simulink model "ModelReadWrite"  (R2016a)
settings: Solver=VariableStepAuto  StartTime=0.0  StopTime=30  RelTol=1e-3
libraries: ToolBox_Control_Lab x1
settings Model: Creator=steph  LastModifiedBy=steph

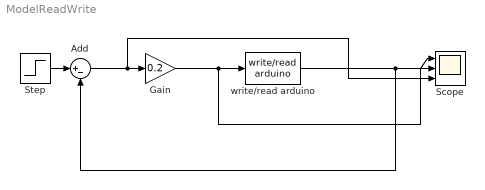
== system ModelReadWrite ==
  Add : Sum  Inputs=|+-
  Gain : Gain  Gain=0.2
  Scope : Scope  NumInputPorts=3
  Step : Step  Time=5  After=23  SampleTime=0
  "write/read arduino " : ToolBox_Control_Lab/write//read arduino    COM='COM9'  MODEL='UNO'  PWM='D9'  SP='A0'  Ts=1
  wires:
  Gain/1 -> "write/read arduino "/1, Scope/2
  Add/1 -> Scope/3, Gain/1
  "write/read arduino "/1 -> Add/2, Scope/1
  Step/1 -> Add/1
